simulink model "power_piline"  (Simulink 6.0)
settings: Solver=ode15s  SolverMode=SingleTasking  StartTime=0.0  StopTime=0.05  RelTol=1e-3  AbsTol=1e-6
libraries: powerlib x10
settings Model: Creator=patrice  LastModifiedBy=batserve  ExtModeTrigMode=oneshot  ExtModeArmWhenConnect=off  ExtModeAutoUpdateStatusClock=off
settings DataIOCC: LimitDataPoints=off  SignalLoggingName=sigsOut
settings OptimizationCC: BooleanDataType=off
settings DebuggingCC: SolverPrmCheckMsg=none
settings HardwareCC: TargetUnknown=on
settings RTWCC: TemplateMakefile=grt_unix.tmf

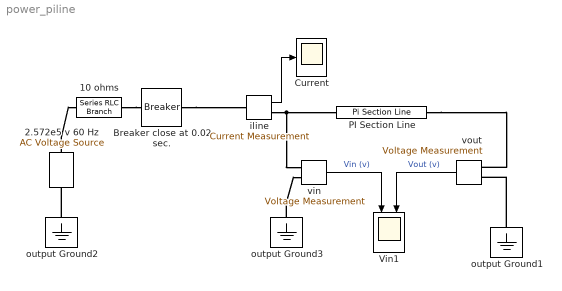
== system power_piline ==
  10 ohms : powerlib/Elements/Series RLC Branch  PhysicalDomain=powersysdomain  SubClassName=unknown  PortType=p1  LConnTagsString=__new0  RConnTagsString=__new0  Resistance=10  Inductance=0  Capacitance=inf  Measurements=None
  "2.572e5 v 60 Hz " : powerlib/Electrical Sources/AC Voltage Source  Description=source block  Orientation=up  Amplitude=(315e3*sqrt(2))/sqrt(30)  Phase=0  Frequency=60  SampleTime=0  Measurements=None
      settings: AttributesFormatString=\n
  Breaker close at 0.02 sec. : powerlib/Elements/Breaker  BreakerResistance=1e-1  InitialState=0  SnubberResistance=inf  SnubberCapacitance=0  SwitchingTimes=[ .02 ]  External=off  Measurements=None
      settings: AttributesFormatString=\n
  Current : Scope
      settings: TickLabels=on  TimeRange=0.05  YMin=-100  YMax=100  DataFormat=Array  MaxDataPoints=5000000
  PI Section Line : powerlib/Elements/Pi Section Line  PhysicalDomain=powersysdomain  SubClassName=unknown  PortType=p1  LConnTagsString=__new0  RConnTagsString=__new0  Frequency=60  Resistance=0.2568  Inductance=2e-03  Capacitance=8.6e-09  Length=100  PiSections=1  Measurements=None
      settings: AttributesFormatString=\n
  Vin1 : Scope  NumInputPorts=2
      settings: Orientation=down  TickLabels=on  TimeRange=0.05  YMin=-100000~-5  YMax=100000~5  DataFormat=Array
  iline : powerlib/Measurements/Current Measurement  Tag=PoWeRsYsTeMmEaSuReMeNt  PhasorSimulation=off  OutputType=Magnitude  PSBequivalent=0
  output Ground1 : powerlib/Elements/Ground  Orientation=down  PhysicalDomain=powersysdomain  SubClassName=unknown  PortType=p1  LConnTagsString=a
  output Ground2 : powerlib/Elements/Ground  Orientation=down  PhysicalDomain=powersysdomain  SubClassName=unknown  PortType=p1  LConnTagsString=a
  output Ground3 : powerlib/Elements/Ground  Orientation=down  PhysicalDomain=powersysdomain  SubClassName=unknown  PortType=p1  LConnTagsString=a
  vin : powerlib/Measurements/Voltage Measurement  Tag=PoWeRsYsTeMmEaSuReMeNt  PhasorSimulation=off  OutputType=Magnitude  PSBequivalent=0
  vout : powerlib/Measurements/Voltage Measurement  Tag=PoWeRsYsTeMmEaSuReMeNt  Orientation=left  PhasorSimulation=off  OutputType=Magnitude  PSBequivalent=0
  wires:
  iline/1 -> Current/1
  vin/1 -> Vin1/1  "Vin (v)"
  vout/1 -> Vin1/2  "Vout (v)"
  connections:
  "2.572e5 v 60 Hz "/RConn1 -- 10 ohms/LConn1
  10 ohms/RConn1 -- Breaker close at 0.02 sec./LConn1
  output Ground2/LConn1 -- "2.572e5 v 60 Hz "/LConn1
  PI Section Line/RConn1 -- vout/LConn1
  output Ground1/LConn1 -- vout/LConn2
  Breaker close at 0.02 sec./RConn1 -- iline/LConn1
  output Ground3/LConn1 -- vin/LConn2
  iline/RConn1 -- PI Section Line/LConn1 -- vin/LConn1
